simulink model "main_program"  (R2024b)
settings: Solver=VariableStepAuto  StartTime=0.0  StopTime=10.0  RelTol=1e-3
InitFcn:
  | initial_param;
  | run('initial_param.m');
undefined symbols (not defined in the file or in its folder): Alloc, Control, Motor, Speed, Vehicle
libraries: simulink x4, slpidlib x1
settings Model: Creator=tomer  LastModifiedBy=tomer

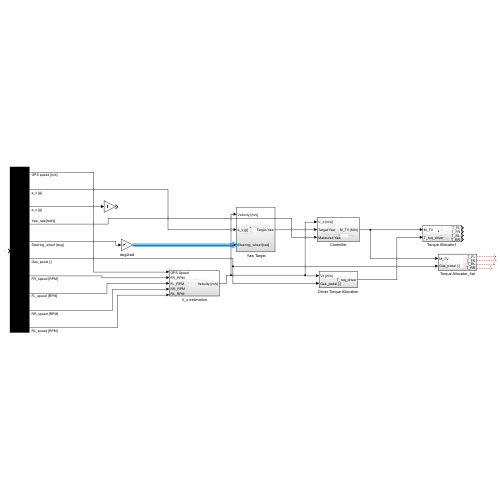
[thumbnail: Simulink's stored preview of the top-level diagram]
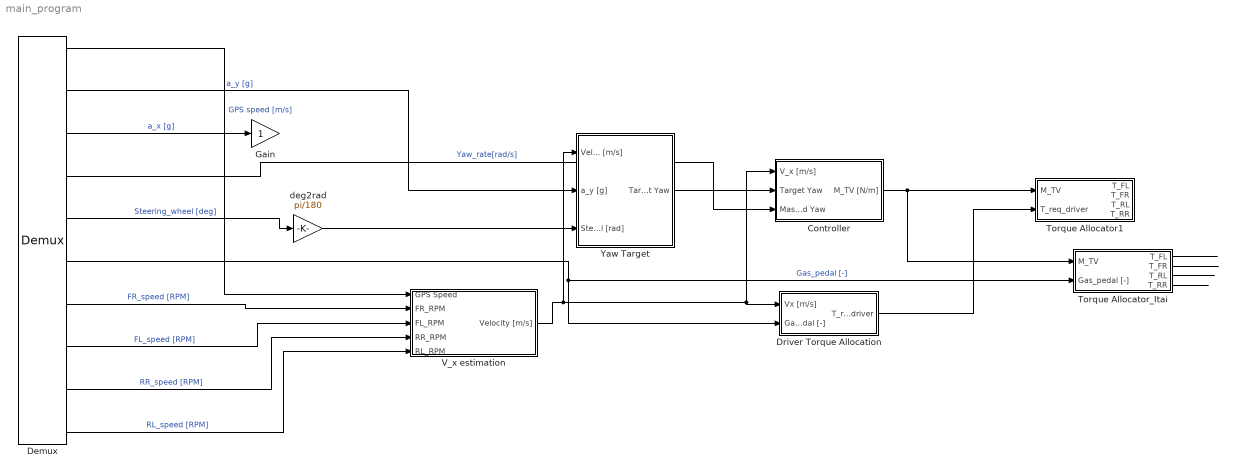
== system main_program ==
  " Yaw Target" : Subsystem
  Controller : Subsystem
  Demux : Demux  Outputs=10
  Driver Torque Allocation : Subsystem
  Gain : Gain
  Torque Allocator1 : Subsystem
  Torque Allocator_Itai : Subsystem
  V_x estimation : Subsystem
  deg2rad : Gain  Gain=pi/180
  wires:
  Demux/1 -> V_x estimation/1(GPS Speed)  "GPS speed [m/s]"
  Demux/2 -> " Yaw Target"/2(a_y [g])  "a_y [g]"
  Demux/3 -> Gain/1  "a_x [g]"
  Demux/4 -> Controller/3(Massured Yaw)  "Yaw_rate[rad/s]"
  Demux/5 -> deg2rad/1  "Steering_wheel [deg]"
  Demux/6 -> Driver Torque Allocation/2(Gas_pedal [-]), Torque Allocator_Itai/2(Gas_pedal [-])  "Gas_pedal [-]"
  Demux/7 -> V_x estimation/2(FR_RPM)  "FR_speed [RPM]"
  Demux/8 -> V_x estimation/3(FL_RPM)  "FL_speed [RPM]"
  Demux/9 -> V_x estimation/4(RR_RPM)  "RR_speed [RPM]"
  Demux/10 -> V_x estimation/5(RL_RPM)  "RL_speed [RPM]"
  " Yaw Target"/1(Target Yaw) -> Controller/2(Target Yaw)
  Controller/1(M_TV [N/m]) -> Torque Allocator1/1(M_TV), Torque Allocator_Itai/1(M_TV)
  Torque Allocator_Itai/4(T_RR) -> ?
  Torque Allocator_Itai/3(T_RL) -> ?
  Torque Allocator_Itai/2(T_FR) -> ?
  Torque Allocator_Itai/1(T_FL) -> ?
  deg2rad/1 -> " Yaw Target"/3(Steering_wheel [rad])
  V_x estimation/1(Velocity [m/s]) -> " Yaw Target"/1(Velocity [m/s]), Driver Torque Allocation/1(Vx [m/s]), Controller/1(V_x [m/s])
  Driver Torque Allocation/1(T_req_driver) -> Torque Allocator1/2(T_req_driver)

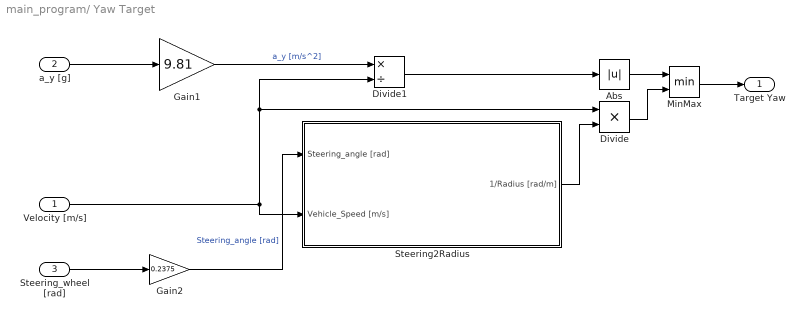
== system main_program/ Yaw Target ==
  Velocity [m/s] : Inport
  a_y [g] : Inport  Port=2
  Steering_wheel [rad] : Inport  Port=3
  Abs : Abs  SaturateOnIntegerOverflow=off
  Divide : Product  Inputs=**
  Divide1 : Product  Inputs=*/
  Gain1 : Gain  Gain=9.81
  Gain2 : Gain  Gain=0.2375
  MinMax : MinMax  Inputs=2
  Steering2Radius : Subsystem
  Target Yaw : Outport
  wires:
  a_y [g]/1 -> Gain1/1
  Velocity [m/s]/1 -> Steering2Radius/2(Vehicle_Speed [m/s]), Divide/1, Divide1/2
  Steering_wheel [rad]/1 -> Gain2/1
  Steering2Radius/1(1/Radius [rad/m]) -> Divide/2
  Gain2/1 -> Steering2Radius/1(Steering_angle [rad])  "Steering_angle [rad]"
  Gain1/1 -> Divide1/1  "a_y [m/s^2]"
  Divide1/1 -> Abs/1
  Abs/1 -> MinMax/1
  Divide/1 -> MinMax/2
  MinMax/1 -> Target Yaw/1

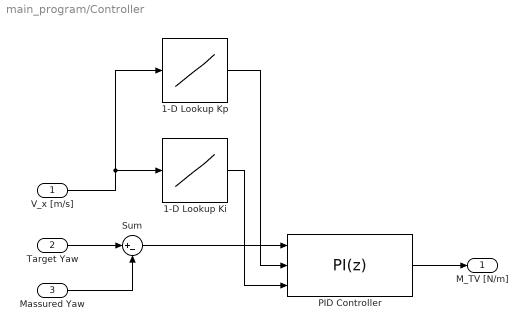
== system main_program/Controller ==
  V_x [m/s] : Inport
  Target Yaw : Inport  Port=2
  Massured Yaw : Inport  Port=3
  1-D Lookup Ki : Lookup_n-D  NumberOfTableDimensions=1  BreakpointsForDimension1=Control.vel_breakpoints  Table=Control.Ki_table  InternalRulePriority=Speed  RndMeth=Simplest
  1-D Lookup Kp : Lookup_n-D  NumberOfTableDimensions=1  BreakpointsForDimension1=Control.vel_breakpoints  Table=Control.Kp_table  InternalRulePriority=Speed  RndMeth=Simplest
  PID Controller : slpidlib/PID Controller  Controller=PI  Form=Parallel  TimeDomain=Discrete-time  UseExternalTs=off  SampleTime=Control.Ts  IntegratorMethod=Forward Euler  FilterMethod=Forward Euler  ControllerParametersSource=external  P=1  I=1  UseKiTs=on  D=0  UseExternalDerivativeSource=off  N=100  UseFilter=on  TunerSelectOption=Transfer Function Based (PID Tuner App)  InitialConditionSource=internal  InitialConditionForIntegrator=0  InitialConditionForFilter=0  DifferentiatorICPrevScaledInput=0  ExternalReset=none  TrackingMode=off  Kt=1  LimitOutput=on  SatLimitsSource=internal  UpperSaturationLimit=Control.MaxYawMoment  LowerSaturationLimit=-Control.MaxYawMoment  LinearizeAsGain=on  AntiWindupMode=clamping  Kb=1  LimitIntegrator=off  UpperIntegratorSaturationLimit=inf  LowerIntegratorSaturationLimit=-inf  POutMin=[]  POutMax=[]  IOutMin=[]  IOutMax=[]  DOutMin=[]  DOutMax=[]  NOutMin=[]  NOutMax=[]  SumOutMin=[]  SumOutMax=[]  SaturationOutMin=[]  SaturationOutMax=[]  PParamMin=[]  PParamMax=[]  IParamMin=[]  IParamMax=[]  DParamMin=[]  DParamMax=[]  NParamMin=[]  NParamMax=[]  KbParamMin=[]  KbParamMax=[]  KtParamMin=[]  KtParamMax=[]  KbOutMin=[]  KbOutMax=[]  KtOutMin=[]  KtOutMax=[]  IntegratorOutMin=[]  IntegratorOutMax=[]  FilterOutMin=[]  FilterOutMax=[]  SumI1OutMin=[]  SumI1OutMax=[]  SumI2OutMin=[]  SumI2OutMax=[]  SumI3OutMin=[]  SumI3OutMax=[]  SumI4OutMin=[]  SumI4OutMax=[]  SumDOutMin=[]  SumDOutMax=[]  DifferentiatorOutMin=[]  DifferentiatorOutMax=[]  FilterDiffOutCoefMin=[]  FilterDiffOutCoefMax=[]  ReciprocalOutMin=[]  ReciprocalOutMax=[]  SumDenOutMin=[]  SumDenOutMax=[]  SumNumOutMin=[]  SumNumOutMax=[]  DivideOutMin=[]  DivideOutMax=[]  UdiffTsProdOutMin=[]  UdiffTsProdOutMax=[]  NTsProdOutMin=[]  NTsProdOutMax=[]  UintegralTsProdOutMin=[]  UintegralTsProdOutMax=[]  UngainTsProdOutMin=[]  UngainTsProdOutMax=[]  ClampingZeroOutDataTypeStr=Inherit: Inherit via back propagation  ClampingZeroOutMin=[]  ClampingZeroOutMax=[]  FilterDenConstantOutDataTypeStr=Inherit: Inherit via back propagation  FilterDenConstantOutMin=[]  FilterDenConstantOutMax=[]  PCopyOutDataTypeStr=Inherit: Inherit via back propagation  PCopyOutMin=[]  PCopyOutMax=[]  NCopyOutDataTypeStr=Inherit: Inherit via back propagation  NCopyOutMin=[]  NCopyOutMax=[]  IntegratorContinuousStateAttributes=''  IntegratorStateMustResolveToSignalObject=off  IntegratorRTWStateStorageClass=Auto  FilterContinuousStateAttributes=''  FilterStateMustResolveToSignalObject=off  FilterRTWStateStorageClass=Auto  ParallelPVariant=ExternalParameters  IdealPVariant=Disabled  IVariant=ExternalParameters  DVariant=Disabled  IntegratorVariant=Discrete  SatVariant=Enabled  AWVariant=DiscClampingParallel  PCopyVariant=Disabled  TRVariant=Disabled  FdbkBlocksVariant=Forward  IdealPFdbkVariant=Disabled  SatFdbkVariant=Disabled  DerivativeFilterVariant=Disabled  NVariant=Disabled  NCopyVariant=Disabled_SignalSpec  FilterICVariant=Disabled  IntegratorICVariant=InternalICs  ExternalResetVariant=Disabled  TRSumVariant=Passthrough  SumFdbkVariant=Disabled  SumVariant=Sum_PI  TsampFilterVariant=InternalTs  TsampNgainVariant=Passthrough  TsampIntegralVariant=Disabled_SignalSpec  ExternalSaturationOutDataTypeStr=Inherit: Same as second input  DerivativeSourceVariant=Disabled  PreIntVariant=InternalPreInt
  Sum : Sum  Inputs=|+-
  M_TV [N/m] : Outport
  wires:
  Target Yaw/1 -> Sum/1
  Massured Yaw/1 -> Sum/2
  Sum/1 -> PID Controller/1
  V_x [m/s]/1 -> 1-D Lookup Ki/1, 1-D Lookup Kp/1
  1-D Lookup Kp/1 -> PID Controller/2
  1-D Lookup Ki/1 -> PID Controller/3
  PID Controller/1 -> M_TV [N/m]/1

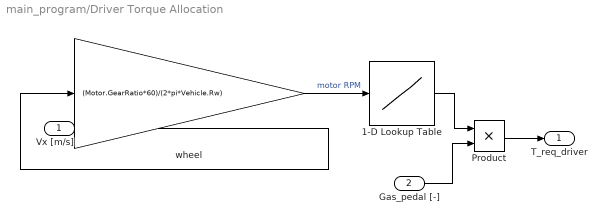
== system main_program/Driver Torque Allocation ==
  Vx [m/s] : Inport
  Gas_pedal [-] : Inport  Port=2
  1-D Lookup Table : Lookup_n-D  NumberOfTableDimensions=1  BreakpointsForDimension1=Motor.RPM_axis  Table=Motor.Torque_axis  InternalRulePriority=Speed  RndMeth=Simplest
  Product : Product
  wheel : Gain  Gain=(Motor.GearRatio*60)/(2*pi*Vehicle.Rw)
  T_req_driver : Outport
  wires:
  Vx [m/s]/1 -> wheel/1
  wheel/1 -> 1-D Lookup Table/1  "motor RPM"
  Product/1 -> T_req_driver/1
  1-D Lookup Table/1 -> Product/1
  Gas_pedal [-]/1 -> Product/2

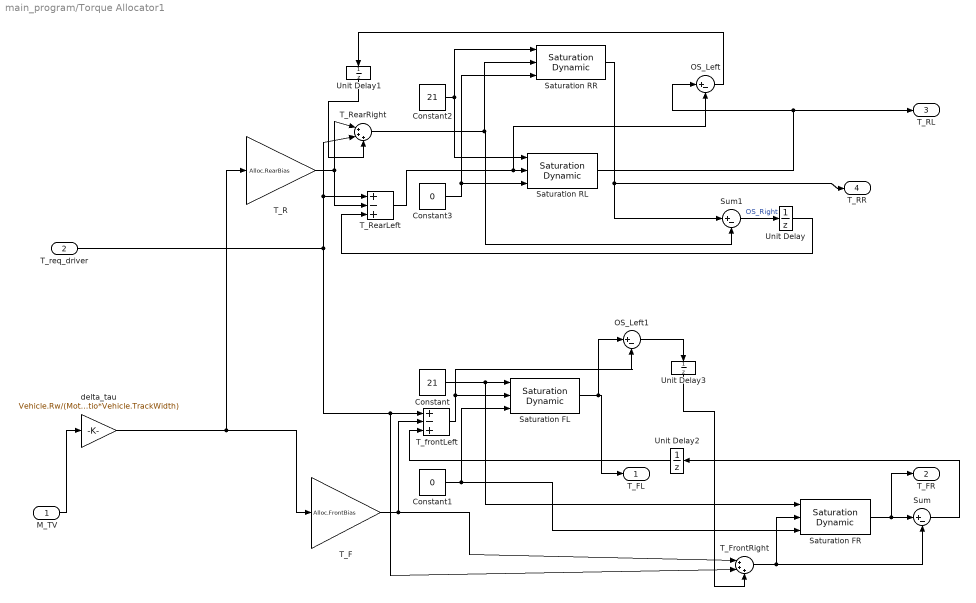
== system main_program/Torque Allocator1 ==
  M_TV : Inport
  T_req_driver : Inport  Port=2
  Constant : Constant  Value=21
  Constant1 : Constant  Value=0
  Constant2 : Constant  Value=21
  Constant3 : Constant  Value=0
  OS_Left : Sum  Inputs=|+-
  OS_Left1 : Sum  Inputs=|+-
  Saturation FL : simulink/Discontinuities/Saturation Dynamic  OutMin=[]  OutMax=[]  OutDataTypeStr=Inherit: Same as second input  OutDataType=fixdt(1, 16)  OutScaling=2^-10  DoSatur=off
  Saturation FR : simulink/Discontinuities/Saturation Dynamic  OutMin=[]  OutMax=[]  OutDataTypeStr=Inherit: Same as second input  OutDataType=fixdt(1, 16)  OutScaling=2^-10  DoSatur=off
  Saturation RL : simulink/Discontinuities/Saturation Dynamic  OutMin=[]  OutMax=[]  OutDataTypeStr=Inherit: Same as second input  OutDataType=fixdt(1, 16)  OutScaling=2^-10  DoSatur=off
  Saturation RR : simulink/Discontinuities/Saturation Dynamic  OutMin=[]  OutMax=[]  OutDataTypeStr=Inherit: Same as second input  OutDataType=fixdt(1, 16)  OutScaling=2^-10  DoSatur=off
  Sum : Sum  Inputs=|+-
  Sum1 : Sum  Inputs=|+-
  T_F : Gain  Gain=Alloc.FrontBias
  T_FrontRight : Sum  Inputs=|+++
  T_R : Gain  Gain=Alloc.RearBias
  T_RearLeft : Sum  Inputs=+-+
  T_RearRight : Sum  Inputs=|+++
  T_frontLeft : Sum  Inputs=+-+
  Unit Delay{,1..3} (4 alike) : UnitDelay  SampleTime=Control.Ts  HasFrameUpgradeWarning=on
  delta_tau : Gain  Gain=Vehicle.Rw/(Motor.GearRatio*Vehicle.TrackWidth)
  T_FL : Outport
  T_FR : Outport  Port=2
  T_RL : Outport  Port=3
  T_RR : Outport  Port=4
  wires:
  T_F/1 -> T_FrontRight/1, T_frontLeft/2
  T_R/1 -> T_RearLeft/2, T_RearRight/1
  M_TV/1 -> delta_tau/1
  T_req_driver/1 -> T_RearRight/2, T_RearLeft/1, T_frontLeft/1, T_FrontRight/2
  delta_tau/1 -> T_F/1, T_R/1
  Unit Delay1/1 -> T_RearRight/3
  Constant2/1 -> Saturation RL/1, Saturation RR/1
  Constant3/1 -> Saturation RR/3, Saturation RL/3
  T_RearRight/1 -> Sum1/2, Saturation RR/2
  Sum1/1 -> Unit Delay/1  "OS_Right"
  Constant/1 -> Saturation FR/1, Saturation FL/1
  T_frontLeft/1 -> OS_Left1/2, Saturation FL/2
  Constant1/1 -> Saturation FL/3, Saturation FR/3
  Saturation RR/1 -> T_RR/1, Sum1/1
  Saturation FL/1 -> T_FL/1, OS_Left1/1
  OS_Left1/1 -> Unit Delay3/1
  Unit Delay3/1 -> T_FrontRight/3
  Unit Delay2/1 -> T_frontLeft/3
  Unit Delay/1 -> T_RearLeft/3
  T_RearLeft/1 -> Saturation RL/2, OS_Left/2
  T_FrontRight/1 -> Sum/2, Saturation FR/2
  Saturation RL/1 -> T_RL/1, OS_Left/1
  Saturation FR/1 -> T_FR/1, Sum/1
  OS_Left/1 -> Unit Delay1/1
  Sum/1 -> Unit Delay2/1

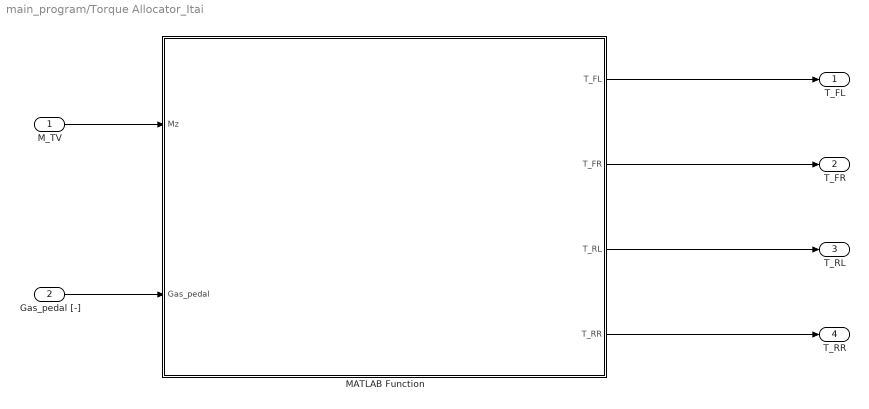
== system main_program/Torque Allocator_Itai ==
  M_TV : Inport
  Gas_pedal [-] : Inport  Port=2
  MATLAB Function : MATLAB Function  TreatAsAtomicUnit=on
  T_FL : Outport
  T_FR : Outport  Port=2
  T_RL : Outport  Port=3
  T_RR : Outport  Port=4
  wires:
  M_TV/1 -> MATLAB Function/1(Mz)
  Gas_pedal [-]/1 -> MATLAB Function/2(Gas_pedal)
  MATLAB Function/1(T_FL) -> T_FL/1
  MATLAB Function/2(T_FR) -> T_FR/1
  MATLAB Function/4(T_RR) -> T_RR/1
  MATLAB Function/3(T_RL) -> T_RL/1

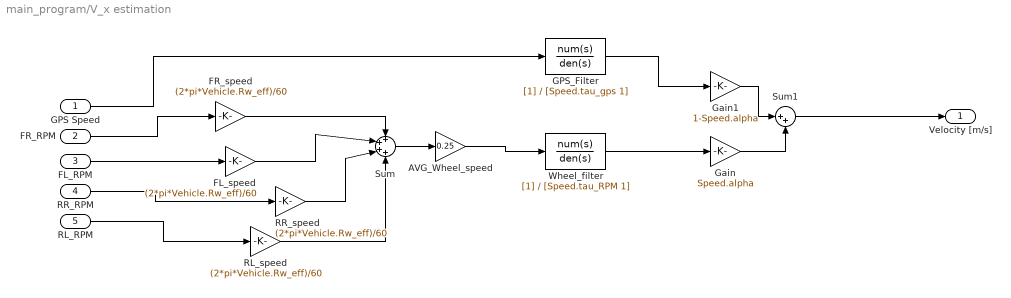
== system main_program/V_x estimation ==
  GPS Speed : Inport
  FR_RPM : Inport  Port=2
  FL_RPM : Inport  Port=3
  RR_RPM : Inport  Port=4
  RL_RPM : Inport  Port=5
  AVG_Wheel_speed : Gain  Gain=0.25
  FL_speed : Gain  Gain=(2*pi*Vehicle.Rw_eff)/60
  FR_speed : Gain  Gain=(2*pi*Vehicle.Rw_eff)/60
  GPS_Filter : TransferFcn  Denominator=[Speed.tau_gps 1]
  Gain : Gain  Gain=Speed.alpha
  Gain1 : Gain  Gain=1-Speed.alpha
  RL_speed : Gain  Gain=(2*pi*Vehicle.Rw_eff)/60
  RR_speed : Gain  Gain=(2*pi*Vehicle.Rw_eff)/60
  Sum : Sum  Inputs=++++
  Sum1 : Sum  Inputs=|++
  Wheel_filter : TransferFcn  Denominator=[Speed.tau_RPM 1]
  Velocity [m/s] : Outport
  wires:
  FR_RPM/1 -> FR_speed/1
  FL_RPM/1 -> FL_speed/1
  RR_RPM/1 -> RR_speed/1
  RL_RPM/1 -> RL_speed/1
  FR_speed/1 -> Sum/1
  FL_speed/1 -> Sum/2
  RR_speed/1 -> Sum/3
  RL_speed/1 -> Sum/4
  Sum/1 -> AVG_Wheel_speed/1
  AVG_Wheel_speed/1 -> Wheel_filter/1
  GPS Speed/1 -> GPS_Filter/1
  Wheel_filter/1 -> Gain/1
  GPS_Filter/1 -> Gain1/1
  Gain1/1 -> Sum1/1
  Gain/1 -> Sum1/2
  Sum1/1 -> Velocity [m/s]/1

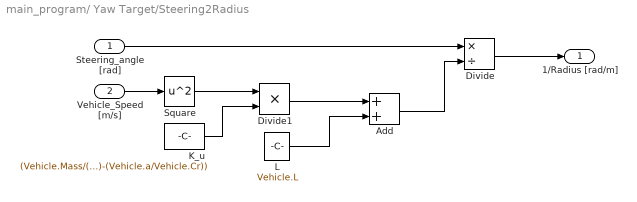
== system main_program/ Yaw Target/Steering2Radius ==
  Steering_angle [rad] : Inport
  Vehicle_Speed [m/s] : Inport  Port=2
  Add : Sum
  Divide : Product  Inputs=*/
  Divide1 : Product  Inputs=**
  K_u : Constant  Value=(Vehicle.Mass/(Vehicle.a+Vehicle.b))*((Vehicle.b/Vehicle.Cf)-(Vehicle.a/Vehicle.Cr))
  L : Constant  Value=Vehicle.L
  Square : Math  Operator=square
  1/Radius [rad/m] : Outport
  wires:
  Steering_angle [rad]/1 -> Divide/1
  Vehicle_Speed [m/s]/1 -> Square/1
  Square/1 -> Divide1/1
  K_u/1 -> Divide1/2
  Divide1/1 -> Add/1
  Add/1 -> Divide/2
  L/1 -> Add/2
  Divide/1 -> 1/Radius [rad/m]/1

== matlab function main_program/Torque Allocator_Itai/MATLAB Function ==
  data: Mz input; T_FL output; Gas_pedal input; T_FR output; T_RL output; T_RR output
%% =========================================================
%  torque_allocator.m
%  BGRacing FSAE - Torque Vectoring Project
%  Tomer Tzahor & Itai Groisman, Ben-Gurion University
%
%  PURPOSE: This is a MATLAB Function block to be placed
%           inside main_program.slx.
%
%  Copy this function body into a MATLAB Function block
%  in Simulink with:
%    Inputs:  Mz [Nm], T_driver [Nm] (base torque demand)
%    Outputs: T_FL, T_FR, T_RL, T_RR [Nm]
%% =========================================================

function [T_FL, T_FR, T_RL, T_RR] = torque_allocator(Mz, Gas_pedal)

%% --- Read parameters from base workspace ---
TrackWidth       = evalin('base', 'Vehicle.TrackWidth');   % [m]
Rw               = evalin('base', 'Vehicle.Rw');           % [m]
MaxWheelTorque   = evalin('base', 'Motor.MaxWheelTorque'); % [Nm]
FrontBias        = evalin('base', 'Alloc.FrontBias');      % [-]
RearBias         = evalin('base', 'Alloc.RearBias');       % [-]

%% --- Base torque demand from driver ---
% Gas_pedal is 0..1, scale to max wheel torque
T_driver = Gas_pedal * MaxWheelTorque;

%% --- Convert Mz to per-axle torque delta ---
% Mz = (ΔF_x) * (TrackWidth/2)
% ΔF_x = Mz / (TrackWidth/2)
% ΔT   = ΔF_x * Rw
delta_T_rear  = (Mz * RearBias)  * Rw / (TrackWidth / 2);
delta_T_front = (Mz * FrontBias) * Rw / (TrackWidth / 2);

%% --- Apply differential torque around base demand ---
% Positive Mz = yaw left = more torque on right wheels
T_RR = T_driver + delta_T_rear  / 2;
T_RL = T_driver - delta_T_rear  / 2;
T_FR = T_driver + delta_T_front / 2;
T_FL = T_driver - delta_T_front / 2;

%% --- Clamp to physical motor limits [0, MaxWheelTorque] ---
T_FL = max(0, min(T_FL, MaxWheelTorque));
T_FR = max(0, min(T_FR, MaxWheelTorque));
T_RL = max(0, min(T_RL, MaxWheelTorque));
T_RR = max(0, min(T_RR, MaxWheelTorque));

end
